simulink model "sampleModel1784"  (R2023a)
settings: Solver=VariableStepAuto  StartTime=0.0  StopTime=10.0  RelTol=1e-3
libraries: hdlsllib x4
settings Model: Creator=user1  LastModifiedBy=user1

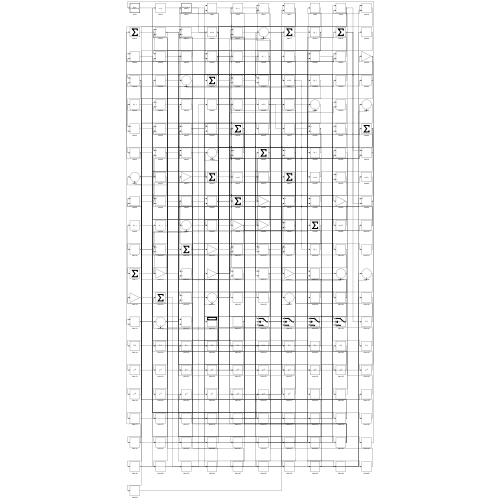
[thumbnail: Simulink's stored preview of the top-level diagram]
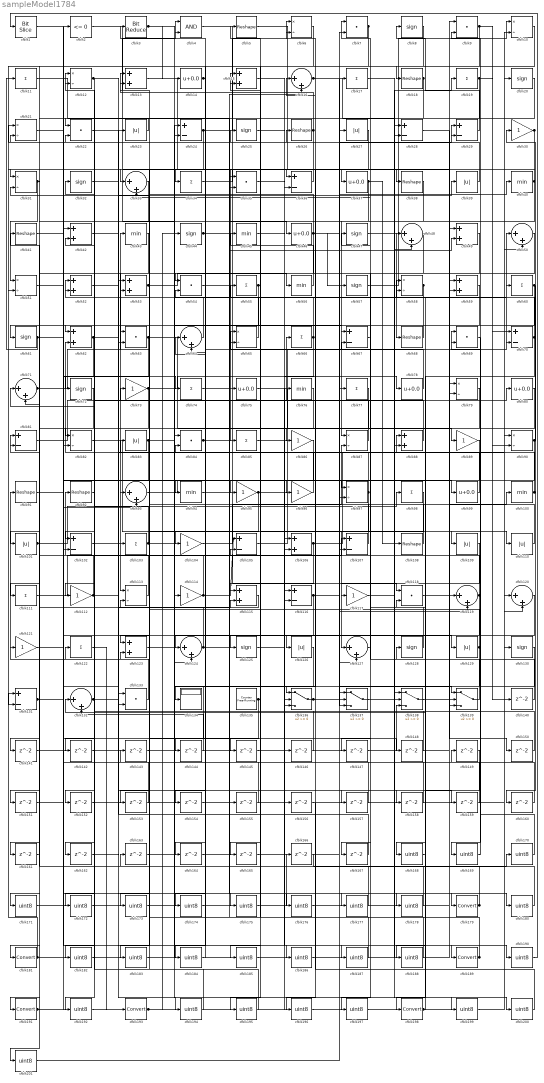
== system sampleModel1784 ==
  cfblk1 : hdlsllib/Logic and Bit Operations/Bit Slice  lidx=7  ridx=0
  cfblk{6,10,12,21,31,51,58,65,79,82,87,90,97,113} (14 alike) : Product  Inputs=*/  RndMeth=Zero  SaturateOnIntegerOverflow=on
  cfblk{40,43,45,56,76,94,100} (7 alike) : MinMax
  cfblk{23,27,39,83,101,109..110,126,129} (9 alike) : Abs  SaturateOnIntegerOverflow=off
  cfblk{24,28..29,36,67,70,81,102,105,107,116,131} (12 alike) : Sum  Inputs=+-
  cfblk{11,17,19,34,55,60,66,74,77,85,98,103,111,122} (14 alike) : Sum  Inputs=+
  cfblk{30,73,86,89,95..96,104,112,114,117,121} (11 alike) : Gain
  cfblk{13,15,42,49,52..53,59,62,88,106,115,123} (12 alike) : Sum
  cfblk{5,18,26,38,41,68,91..92,108} (9 alike) : Reshape
  cfblk{7,9,22,35,54,63,69,84,118,133} (10 alike) : DotProduct  OutDataTypeStr=Inherit: Inherit via internal rule
  cfblk{16,33,48,50,64,71,93,119..120,124,127,132} (12 alike) : Sum  Inputs=|++
  cfblk{8,20,25,32,44,47,57,61,72,125,128,130} (12 alike) : Signum
  cfblk134 : Display
  cfblk135 : hdlsllib/Sources/Counter Free-Running  NumBits=16  tsamp=-1
  cfblk{136..139} (4 alike) : Switch  SaturateOnIntegerOverflow=off  InputSameDT=off
  cfblk{14,37,46,75,78,80,99} (7 alike) : Bias  Bias=0.0  SaturateOnIntegerOverflow=off
  cfblk{140..167} (28 alike) : Delay  SampleTime=1
  cfblk{168..178,180,182..188,190,192,194..197,199..201} (28 alike) : DataTypeConversion  OutDataTypeStr=uint8  SaturateOnIntegerOverflow=off  RndMeth=Floor
  cfblk{179,181,189,191,193,198} (6 alike) : DataTypeConversion  SaturateOnIntegerOverflow=off  RndMeth=Floor
  cfblk2 : hdlsllib/Logic and Bit Operations/Compare To Zero  relop=<=  OutDataTypeStr=boolean
  cfblk3 : hdlsllib/Logic and Bit Operations/Bit Reduce  mode=AND
  cfblk4 : Logic  AllPortsSameDT=off  OutDataTypeStr=boolean
  wires:
  cfblk12/1 -> cfblk72/1, cfblk157/1, cfblk158/1
  cfblk97/1 -> cfblk127/1, cfblk15/2
  cfblk128/1 -> cfblk7/1
  cfblk47/1 -> cfblk68/1
  cfblk68/1 -> cfblk62/1
  cfblk73/1 -> cfblk78/1, cfblk93/1
  cfblk13/1 -> cfblk37/1
  cfblk53/1 -> cfblk56/1, cfblk67/1
  cfblk133/1 -> cfblk91/1
  cfblk88/1 -> cfblk66/1
  cfblk105/1 -> cfblk50/1
  cfblk31/1 -> cfblk51/1, cfblk171/1
  cfblk62/1 -> cfblk82/2, cfblk178/1
  cfblk37/1 -> cfblk87/1, cfblk108/1
  cfblk43/1 -> cfblk113/1
  cfblk57/1 -> cfblk10/1
  cfblk56/1 -> cfblk4/1
  cfblk55/1 -> cfblk164/1, cfblk165/1
  cfblk101/1 -> cfblk98/1, cfblk129/1
  cfblk3/1 -> cfblk14/1, cfblk199/1
  cfblk80/1 -> cfblk132/1
  cfblk2/1 -> cfblk38/1
  cfblk44/1 -> cfblk118/1, cfblk46/1
  cfblk19/1 -> cfblk90/2, cfblk140/1, cfblk141/1
  cfblk92/1 -> cfblk52/1
  cfblk10/1 -> cfblk61/1
  cfblk119/1 -> cfblk126/1, cfblk63/1
  cfblk112/1 -> cfblk92/1, cfblk115/2
  cfblk9/1 -> cfblk18/1, cfblk51/2, cfblk70/1
  cfblk34/1 -> cfblk36/1
  cfblk99/1 -> cfblk62/2
  cfblk122/1 -> cfblk193/1
  cfblk85/1 -> cfblk20/1
  cfblk93/1 -> cfblk95/1
  cfblk65/1 -> cfblk52/2
  cfblk63/1 -> cfblk86/1, cfblk152/1
  cfblk4/1 -> cfblk138/1
  cfblk110/1 -> cfblk5/1
  cfblk51/1 -> cfblk74/1
  cfblk36/1 -> cfblk31/1
  cfblk106/1 -> cfblk28/1, cfblk125/1
  cfblk123/1 -> cfblk24/1
  cfblk78/1 -> cfblk3/1
  cfblk104/1 -> cfblk87/2
  cfblk115/1 -> cfblk113/2
  cfblk49/1 -> cfblk111/1
  cfblk25/1 -> cfblk106/1
  cfblk30/1 -> cfblk123/1, cfblk136/1
  cfblk6/1 -> cfblk54/1
  cfblk81/1 -> cfblk80/1
  cfblk129/1 -> cfblk58/1, cfblk83/1, cfblk137/3
  cfblk7/1 -> cfblk24/2, cfblk185/1
  cfblk117/1 -> cfblk19/1
  cfblk27/1 -> cfblk85/1
  cfblk61/1 -> cfblk11/1, cfblk99/1
  cfblk14/1 -> cfblk124/1, cfblk134/1
  cfblk18/1 -> cfblk36/2, cfblk34/1
  cfblk100/1 -> cfblk47/1, cfblk69/1
  cfblk107/1 -> cfblk65/1
  cfblk87/1 -> cfblk42/2
  cfblk109/1 -> cfblk117/1
  cfblk54/1 -> cfblk58/2
  cfblk135/1 -> cfblk65/2, cfblk183/1
  cfblk23/1 -> cfblk22/1
  cfblk5/1 -> cfblk119/1
  cfblk102/1 -> cfblk103/1
  cfblk71/1 -> cfblk43/1, cfblk96/1, cfblk101/1
  cfblk118/1 -> cfblk100/1
  cfblk46/1 -> cfblk57/1, cfblk29/2, cfblk25/1, cfblk153/1
  cfblk21/1 -> cfblk133/2
  cfblk70/1 -> cfblk15/1, cfblk188/1
  cfblk111/1 -> cfblk107/1
  cfblk15/1 -> cfblk116/1
  cfblk132/1 -> cfblk39/1, cfblk88/1
  cfblk29/1 -> cfblk8/1
  cfblk22/1 -> cfblk124/2
  cfblk121/1 -> cfblk179/1
  cfblk137/1 -> cfblk29/1
  cfblk16/1 -> cfblk28/2, cfblk139/1
  cfblk72/1 -> cfblk82/1
  cfblk114/1 -> cfblk105/1, cfblk32/1, cfblk69/2, cfblk16/2
  cfblk24/1 -> cfblk6/1, cfblk88/2, cfblk63/2
  cfblk77/1 -> cfblk191/1
  cfblk35/1 -> cfblk97/1
  cfblk138/1 -> cfblk9/1
  cfblk130/1 -> cfblk198/1
  cfblk136/1 -> cfblk27/1, cfblk119/2, cfblk70/2
  cfblk40/1 -> cfblk33/1, cfblk201/1
  cfblk103/1 -> cfblk12/1, cfblk60/1, cfblk159/1
  cfblk20/1 -> cfblk102/1
  cfblk58/1 -> cfblk104/1, cfblk142/1
  cfblk131/1 -> cfblk93/2, cfblk145/1
  cfblk39/1 -> cfblk21/2
  cfblk64/1 -> cfblk53/2
  cfblk66/1 -> cfblk55/1, cfblk106/2
  cfblk108/1 -> cfblk31/2
  cfblk124/1 -> cfblk71/2, cfblk67/2, cfblk137/2
  cfblk60/1 -> cfblk160/1, cfblk161/1, cfblk162/1
  cfblk84/1 -> cfblk49/2, cfblk180/1
  cfblk113/1 -> cfblk81/1
  cfblk38/1 -> cfblk112/1
  cfblk52/1 -> cfblk23/1
  cfblk75/1 -> cfblk89/1
  cfblk11/1 -> cfblk75/1
  cfblk26/1 -> cfblk13/1, cfblk131/2, cfblk192/1
  cfblk1/1 -> cfblk189/1
  cfblk48/1 -> cfblk181/1
  cfblk90/1 -> cfblk30/1, cfblk139/3
  cfblk96/1 -> cfblk12/2
  cfblk83/1 -> cfblk102/2, cfblk139/2
  cfblk139/1 -> cfblk33/2
  cfblk98/1 -> cfblk115/1
  cfblk8/1 -> cfblk94/1
  cfblk95/1 -> cfblk50/2, cfblk173/1
  cfblk82/1 -> cfblk110/1
  cfblk116/1 -> cfblk40/1, cfblk154/1
  cfblk74/1 -> cfblk109/1
  cfblk89/1 -> cfblk116/2
  cfblk140/1 -> cfblk21/1
  cfblk141/1 -> cfblk107/2
  cfblk143/1 -> cfblk7/2
  cfblk126/1 -> cfblk144/1
  cfblk144/1 -> cfblk132/2
  cfblk145/1 -> cfblk138/3
  cfblk146/1 -> cfblk64/1
  cfblk50/1 -> cfblk147/1
  cfblk147/1 -> cfblk49/1
  cfblk32/1 -> cfblk148/1
  cfblk148/1 -> cfblk71/1
  cfblk28/1 -> cfblk150/1
  cfblk150/1 -> cfblk138/2
  cfblk33/1 -> cfblk151/1
  cfblk152/1 -> cfblk35/2
  cfblk153/1 -> cfblk22/2
  cfblk154/1 -> cfblk90/1
  cfblk94/1 -> cfblk155/1
  cfblk155/1 -> cfblk53/1
  cfblk125/1 -> cfblk156/1
  cfblk157/1 -> cfblk42/1
  cfblk158/1 -> cfblk4/2
  cfblk159/1 -> cfblk6/2
  cfblk160/1 -> cfblk123/2
  cfblk161/1 -> cfblk81/2
  cfblk163/1 -> cfblk84/1
  cfblk164/1 -> cfblk127/2
  cfblk165/1 -> cfblk97/2
  cfblk67/1 -> cfblk167/1
  cfblk167/1 -> cfblk133/1
  cfblk149/1 -> cfblk168/1
  cfblk168/1 -> cfblk118/2
  cfblk69/1 -> cfblk169/1
  cfblk169/1 -> cfblk149/1
  cfblk166/1 -> cfblk170/1
  cfblk170/1 -> cfblk9/2
  cfblk171/1 -> cfblk166/1
  cfblk76/1 -> cfblk172/1
  cfblk172/1 -> cfblk146/1
  cfblk173/1 -> cfblk76/1
  cfblk59/1 -> cfblk174/1
  cfblk174/1 -> cfblk64/2
  cfblk91/1 -> cfblk175/1
  cfblk175/1 -> cfblk59/1
  cfblk151/1 -> cfblk176/1
  cfblk176/1 -> cfblk59/2
  cfblk41/1 -> cfblk177/1
  cfblk177/1 -> cfblk143/1
  cfblk178/1 -> cfblk41/1
  cfblk179/1 -> cfblk136/2, cfblk54/2
  cfblk180/1 -> cfblk121/1
  cfblk181/1 -> cfblk114/1, cfblk131/1
  cfblk86/1 -> cfblk182/1
  cfblk182/1 -> cfblk48/1
  cfblk183/1 -> cfblk48/2
  cfblk79/1 -> cfblk184/1
  cfblk184/1 -> cfblk84/2
  cfblk185/1 -> cfblk79/1
  cfblk142/1 -> cfblk186/1
  cfblk186/1 -> cfblk79/2
  cfblk45/1 -> cfblk187/1
  cfblk187/1 -> cfblk163/1
  cfblk188/1 -> cfblk45/1
  cfblk189/1 -> cfblk13/2, cfblk26/1, cfblk105/2, cfblk35/1
  cfblk162/1 -> cfblk190/1
  cfblk190/1 -> cfblk1/1
  cfblk191/1 -> cfblk2/1, cfblk137/1
  cfblk192/1 -> cfblk77/1
  cfblk193/1 -> cfblk136/3, cfblk44/1
  cfblk42/1 -> cfblk194/1
  cfblk194/1 -> cfblk122/1
  cfblk120/1 -> cfblk195/1
  cfblk195/1 -> cfblk73/1
  cfblk156/1 -> cfblk196/1
  cfblk196/1 -> cfblk120/1
  cfblk127/1 -> cfblk197/1
  cfblk197/1 -> cfblk120/2
  cfblk198/1 -> cfblk10/2, cfblk128/1
  cfblk199/1 -> cfblk130/1
  cfblk17/1 -> cfblk200/1
  cfblk200/1 -> cfblk16/1
  cfblk201/1 -> cfblk17/1
